simulink library "csc_ppc_phase_plane_ctrl_lib"  (R2015b)
settings: Solver=ode45  SolverMode=SingleTasking  StartTime=0.0  StopTime=10.0  RelTol=1e-3
libraries: util_quat_lib x2, util_info_lib x1, util_common_lib x1, csc_cac_coarse_acs_ctrl_lib x1, csc_vac_gimbal_steering_vernier_roll_acs_ctrl_lib_diag x1, csc_vac_vernier_acs_ctrl_lib x1
settings Model: ExtModeAutoUpdateStatusClock=off  Creator=nvk  LastModifiedBy=jimkaidy
settings DataIOCC: SaveFormat=Array  SignalLoggingSaveFormat=ModelDataLogs
settings OptimizationCC: BlockReduction=off  BooleanDataType=off
settings DebuggingCC: SaveWithParameterizedLinksMsg=none  UnderspecifiedInitializationDetection=Classic  MergeDetectMultiDrivingBlocksExec=none  SignalResolutionControl=TryResolveAllWithWarning  StateNameClashWarn=warning  StrictBusMsg=Warning
settings HardwareCC: ProdBitPerPointer=32  ProdLargestAtomicFloat=None  ProdIntDivRoundTo=Undefined  ProdEndianess=Unspecified  ProdWordSize=32  ProdHWDeviceType=32-bit Generic  TargetUnknown=on
settings GRTTargetCC: GeneratePreprocessorConditionals=Disable all
settings ConfigComp: CovModelRefEnable=Off  CovSFcnEnable=off

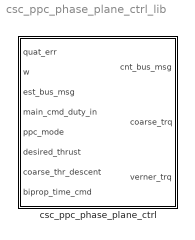
== system csc_ppc_phase_plane_ctrl_lib ==
  csc_ppc_phase_plane_ctrl : Subsystem

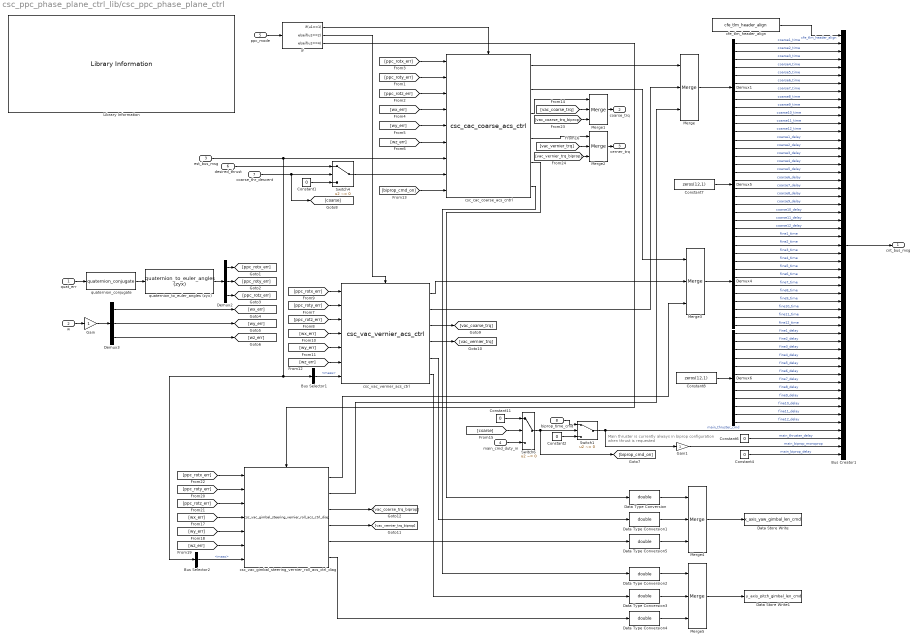
== system csc_ppc_phase_plane_ctrl_lib/csc_ppc_phase_plane_ctrl ==
  note: Main thruster is currently always in biprop configuration
      | when thrust is requested
  quat_err : Inport
  w : Inport  Port=2
  est_bus_msg : Inport  Port=3
  main_cmd_duty_in : Inport  Port=4
  ppc_mode : Inport  Port=5
  desired_thrust : Inport  Port=6
  coarse_thr_descent : Inport  Port=7
  biprop_time_cmd : Inport  Port=8
  Bus Creator1 : BusCreator  Inputs=53  OutDataTypeStr=Bus: cnt_bus_msg  NonVirtualBus=on
  Bus Selector1 : BusSelector  OutputSignals=mass
  Bus Selector2 : BusSelector  OutputSignals=mass
  Constant1 : Constant  Value=0
  Constant11 : Constant  Value=0  OutDataTypeStr=boolean
  Constant2 : Constant  Value=0  OutDataTypeStr=uint8
  Constant4 : Constant  Value=0  OutDataTypeStr=uint8
  Constant6 : Constant  Value=0  OutDataTypeStr=uint8
  Constant7 : Constant  Value=zeros(12,1)  OutDataTypeStr=uint8
  Constant8 : Constant  Value=zeros(12,1)  OutDataTypeStr=uint8
  Data Store Write : DataStoreWrite  DataStoreName=y_axis_yaw_gimbal_len_cmd  DataStoreElements=x_axis_yaw_gimbal_len_cmd
  Data Store Write1 : DataStoreWrite  DataStoreName=x_axis_pitch_gimbal_len_cmd  DataStoreElements=y_axis_pitch_gimbal_len_cmd
  Data Type Conversion{,1..5} (6 alike) : DataTypeConversion  OutDataTypeStr=double
  Demux{1,4..6} (4 alike) : Demux  Outputs=12
  Demux2 : Demux  Outputs=3
  Demux3 : Demux  Outputs=3
  Gain : Gain
  Gain1 : Gain  OutDataTypeStr=uint8
  If : If  IfExpression=u1==1  ElseIfExpressions=u1==2,u1==4  ShowElse=off
  Library Information : util_info_lib/Library Information  owner='jkaidy'
  Merge{,1..3} (4 alike) : Merge  Inputs=3
  Merge4 : Merge  Inputs=3  InitialOutput=0
  Merge5 : Merge  Inputs=3  InitialOutput=0
  Switch1 : Switch  Criteria=u2 ~= 0
  Switch4 : Switch  Criteria=u2 ~= 0
  Switch6 : Switch  Criteria=u2 ~= 0
  cfe_tlm_header_align : util_common_lib/cfe_tlm_header_align
  csc_cac_coarse_acs_cntrl : csc_cac_coarse_acs_ctrl_lib/csc_cac_coarse_acs_ctrl
  csc_vac_gimbal_steering_vernier_roll_acs_ctrl_diag : csc_vac_gimbal_steering_vernier_roll_acs_ctrl_lib_diag/csc_vac_gimbal_steering_vernier_roll_acs_ctrl_diag
  csc_vac_vernier_acs_ctrl : csc_vac_vernier_acs_ctrl_lib/csc_vac_vernier_acs_ctrl
  quaternion_conjugate : util_quat_lib/quaternion_conjugate  SystemSampleTime=-1
  quaternion_to_euler_angles (zyx) : util_quat_lib/quaternion_to_euler_angles (zyx)  SystemSampleTime=-1
  cnt_bus_msg : Outport
  coarse_trq : Outport  Port=2
  verner_trq : Outport  Port=3
  wires:
  Gain1/1 -> Bus Creator1/52  "main_biprop_monoprop"
  csc_vac_vernier_acs_ctrl/2 -> Merge/2
  csc_vac_vernier_acs_ctrl/1 -> Merge3/2
  Constant8/1 -> Demux6/1
  Constant7/1 -> Demux5/1
  Demux6/11 -> Bus Creator1/48  "fine11_delay"
  Demux6/7 -> Bus Creator1/44  "fine7_delay"
  Demux6/12 -> Bus Creator1/49  "fine12_delay"
  Demux6/2 -> Bus Creator1/39  "fine2_delay"
  Demux6/5 -> Bus Creator1/42  "fine5_delay"
  Demux6/8 -> Bus Creator1/45  "fine8_delay"
  Demux6/3 -> Bus Creator1/40  "fine3_delay"
  Demux6/6 -> Bus Creator1/43  "fine6_delay"
  Demux6/9 -> Bus Creator1/46  "fine9_delay"
  Demux6/4 -> Bus Creator1/41  "fine4_delay"
  Demux6/10 -> Bus Creator1/47  "fine10_delay"
  Demux6/1 -> Bus Creator1/38  "fine1_delay"
  Constant6/1 -> Bus Creator1/51  "main_thruster_delay"
  Constant4/1 -> Bus Creator1/53  "main_biprop_delay"
  Demux4/11 -> Bus Creator1/36  "fine11_time"
  Demux4/6 -> Bus Creator1/31  "fine6_time"
  Demux4/3 -> Bus Creator1/28  "fine3_time"
  Demux4/12 -> Bus Creator1/37  "fine12_time"
  Demux4/5 -> Bus Creator1/30  "fine5_time"
  Demux4/1 -> Bus Creator1/26  "fine1_time"
  Demux4/2 -> Bus Creator1/27  "fine2_time"
  Demux4/7 -> Bus Creator1/32  "fine7_time"
  Demux4/8 -> Bus Creator1/33  "fine8_time"
  Demux4/10 -> Bus Creator1/35  "fine10_time"
  Demux4/9 -> Bus Creator1/34  "fine9_time"
  Demux4/4 -> Bus Creator1/29  "fine4_time"
  Demux5/10 -> Bus Creator1/23  "coarse10_delay"
  Demux5/7 -> Bus Creator1/20  "coarse7_delay"
  Demux5/11 -> Bus Creator1/24  "coarse11_delay"
  Demux5/1 -> Bus Creator1/14  "coarse1_delay"
  Demux5/5 -> Bus Creator1/18  "coarse5_delay"
  Demux5/9 -> Bus Creator1/22  "coarse9_delay"
  Demux5/12 -> Bus Creator1/25  "coarse12_delay"
  Demux5/2 -> Bus Creator1/15  "coarse2_delay"
  Demux5/8 -> Bus Creator1/21  "coarse8_delay"
  Demux5/6 -> Bus Creator1/19  "coarse6_delay"
  Demux5/4 -> Bus Creator1/17  "coarse4_delay"
  Demux5/3 -> Bus Creator1/16  "coarse3_delay"
  Merge3/1 -> Demux4/1
  Demux1/11 -> Bus Creator1/12  "coarse11_time"
  Demux1/2 -> Bus Creator1/3  "coarse2_time"
  Demux1/10 -> Bus Creator1/11  "coarse10_time"
  Demux1/5 -> Bus Creator1/6  "coarse5_time"
  Demux1/3 -> Bus Creator1/4  "coarse3_time"
  Demux1/6 -> Bus Creator1/7  "coarse6_time"
  Demux1/4 -> Bus Creator1/5  "coarse4_time"
  Demux1/7 -> Bus Creator1/8  "coarse7_time"
  Demux1/12 -> Bus Creator1/13  "coarse12_time"
  Demux1/9 -> Bus Creator1/10  "coarse9_time"
  Demux1/8 -> Bus Creator1/9  "coarse8_time"
  Demux1/1 -> Bus Creator1/2  "coarse1_time"
  Merge/1 -> Demux1/1
  csc_cac_coarse_acs_cntrl/2 -> Merge3/1
  csc_vac_vernier_acs_ctrl/4 -> [vac_vernier_trq]
  cfe_tlm_header_align/1 -> Bus Creator1/1  "cfe_tlm_header_align"
  [vac_vernier_trq] -> Merge2/2
  [vac_coarse_trq] -> Merge1/2
  csc_vac_vernier_acs_ctrl/3 -> [vac_coarse_trq]
  csc_cac_coarse_acs_cntrl/4 -> Merge2/1
  csc_cac_coarse_acs_cntrl/3 -> Merge1/1
  Merge1/1 -> coarse_trq/1
  If/2 -> csc_vac_vernier_acs_ctrl/Action
  If/1 -> csc_cac_coarse_acs_cntrl/Action
  ppc_mode/1 -> If/1
  Demux2/2 -> [ppc_roty_err]
  Demux2/3 -> [ppc_rotz_err]
  Demux2/1 -> [ppc_rotx_err]
  quaternion_conjugate/1 -> quaternion_to_euler_angles (zyx)/1
  quaternion_to_euler_angles (zyx)/1 -> Demux2/1
  Bus Creator1/1 -> cnt_bus_msg/1
  Switch1/1 -> Gain1/1, Bus Creator1/50  "main_thruster_cmd"
  coarse_thr_descent/1 -> Switch4/2, [coarse]
  Switch4/1 -> csc_cac_coarse_acs_cntrl/8
  desired_thrust/1 -> Switch4/1
  Constant1/1 -> Switch4/3
  Switch6/1 -> [biprop_cmd_on], Switch1/2
  Constant11/1 -> Switch6/1
  main_cmd_duty_in/1 -> Switch6/3
  [coarse] -> Switch6/2
  Constant2/1 -> Switch1/3
  biprop_time_cmd/1 -> Switch1/1
  quat_err/1 -> quaternion_conjugate/1
  w/1 -> Gain/1
  [ppc_rotz_err] -> csc_cac_coarse_acs_cntrl/3
  [wy_err] -> csc_cac_coarse_acs_cntrl/5
  [wx_err] -> csc_cac_coarse_acs_cntrl/4
  [ppc_rotx_err] -> csc_cac_coarse_acs_cntrl/1
  [ppc_roty_err] -> csc_cac_coarse_acs_cntrl/2
  [wz_err] -> csc_cac_coarse_acs_cntrl/6
  [wy_err] -> csc_vac_vernier_acs_ctrl/5
  [wx_err] -> csc_vac_vernier_acs_ctrl/4
  [wz_err] -> csc_vac_vernier_acs_ctrl/6
  [ppc_rotz_err] -> csc_vac_vernier_acs_ctrl/3
  [ppc_roty_err] -> csc_vac_vernier_acs_ctrl/2
  [ppc_rotx_err] -> csc_vac_vernier_acs_ctrl/1
  est_bus_msg/1 -> Bus Selector2/1, Bus Selector1/1, csc_cac_coarse_acs_cntrl/7
  Gain/1 -> Demux3/1
  Demux3/1 -> [wx_err]
  Demux3/2 -> [wy_err]
  Demux3/3 -> [wz_err]
  csc_cac_coarse_acs_cntrl/1 -> Merge/1
  Bus Selector1/1 -> csc_vac_vernier_acs_ctrl/7  "<mass>"
  [biprop_cmd_on] -> csc_cac_coarse_acs_cntrl/9
  Bus Selector2/1 -> csc_vac_gimbal_steering_vernier_roll_acs_ctrl_diag/7  "<mass>"
  [wy_err] -> csc_vac_gimbal_steering_vernier_roll_acs_ctrl_diag/5
  [wx_err] -> csc_vac_gimbal_steering_vernier_roll_acs_ctrl_diag/4
  [wz_err] -> csc_vac_gimbal_steering_vernier_roll_acs_ctrl_diag/6
  [ppc_rotz_err] -> csc_vac_gimbal_steering_vernier_roll_acs_ctrl_diag/3
  [ppc_roty_err] -> csc_vac_gimbal_steering_vernier_roll_acs_ctrl_diag/2
  [ppc_rotx_err] -> csc_vac_gimbal_steering_vernier_roll_acs_ctrl_diag/1
  csc_vac_gimbal_steering_vernier_roll_acs_ctrl_diag/4 -> [vac_vernier_trq_biprop]
  csc_vac_gimbal_steering_vernier_roll_acs_ctrl_diag/3 -> [vac_coarse_trq_biprop]
  If/3 -> csc_vac_gimbal_steering_vernier_roll_acs_ctrl_diag/Action
  csc_vac_gimbal_steering_vernier_roll_acs_ctrl_diag/1 -> Merge3/3
  csc_vac_gimbal_steering_vernier_roll_acs_ctrl_diag/2 -> Merge/3
  [vac_vernier_trq_biprop] -> Merge2/3
  [vac_coarse_trq_biprop] -> Merge1/3
  Merge2/1 -> verner_trq/1
  Merge4/1 -> Data Store Write/1
  Merge5/1 -> Data Store Write1/1
  csc_vac_gimbal_steering_vernier_roll_acs_ctrl_diag/6 -> Data Type Conversion4/1
  csc_vac_gimbal_steering_vernier_roll_acs_ctrl_diag/5 -> Data Type Conversion5/1
  csc_cac_coarse_acs_cntrl/5 -> Data Type Conversion/1
  Data Type Conversion/1 -> Merge4/1
  Data Type Conversion1/1 -> Merge4/2
  Data Type Conversion2/1 -> Merge5/1
  Data Type Conversion3/1 -> Merge5/2
  Data Type Conversion4/1 -> Merge5/3
  Data Type Conversion5/1 -> Merge4/3
  csc_vac_vernier_acs_ctrl/6 -> Data Type Conversion3/1
  csc_cac_coarse_acs_cntrl/6 -> Data Type Conversion2/1
  csc_vac_vernier_acs_ctrl/5 -> Data Type Conversion1/1
